simulink subsystem "rigid_body_sixdof"  (R2024b)
settings: Solver=VariableStepAuto  StartTime=0.0  StopTime=10.0  RelTol=1e-3
model mask{pos_0=[0; 0; 0], vel_0=[0; 0; 0], ornt_0=[1; 0; 0; 0], mass=1, inertia=eye(2), spin_0=[0; 0; 0]}
  mask prompts: pos_0 "Initial position, inertial [m]"; vel_0 "Initial velocity, inertial [m/s]"; ornt_0 "Initial orientation [quat]"; mass "Constant mass"; inertia "Rotational inertia, body coordinates"; spin_0 "Initial spin [rad/s]"
settings Model: Creator=yevge  LastModifiedBy=Yevgeniy Gorbachev

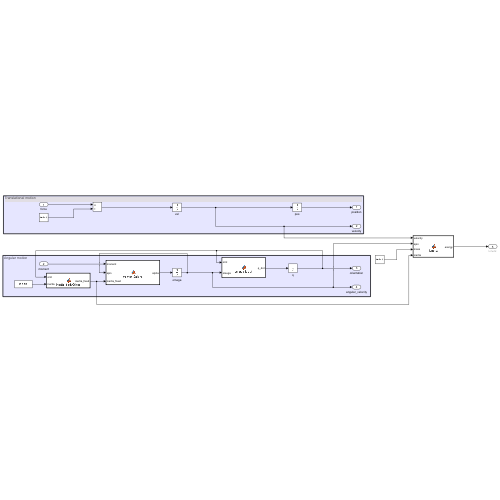
[thumbnail: Simulink's stored preview of the top-level diagram]
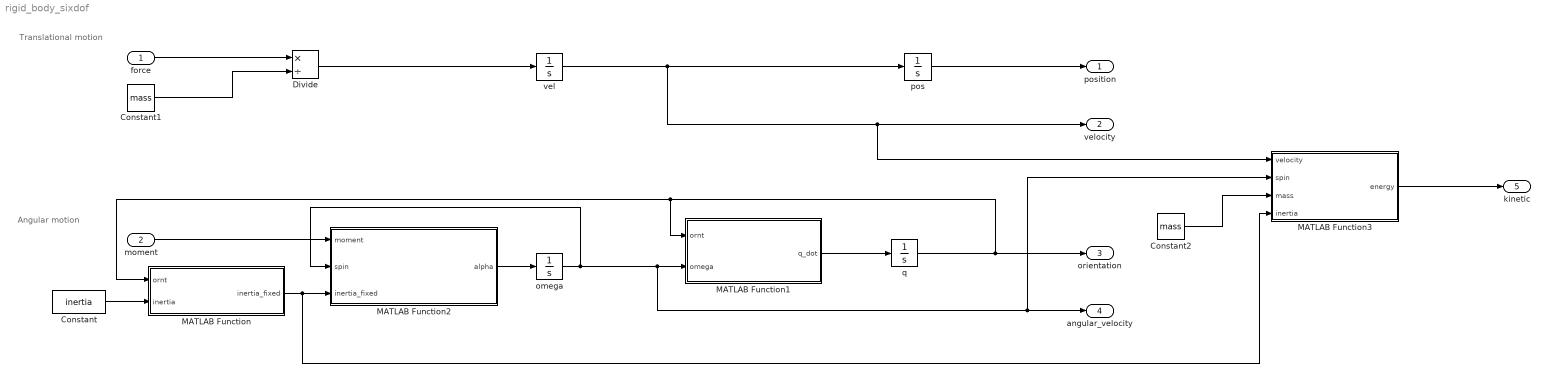
== system rigid_body_sixdof ==
  note: Angular motion
  note: Translational motion
  force : Inport  Unit=N  PortDimensions=[3 1]
  moment : Inport  Port=2  Unit=N*m@torque  PortDimensions=[3 1]
  Constant : Constant  Value=inertia
  Constant1 : Constant  Value=mass
  Constant2 : Constant  Value=mass
  Divide : Product  Inputs=*/
  MATLAB Function : MATLAB Function  TreatAsAtomicUnit=on
  MATLAB Function1 : MATLAB Function  TreatAsAtomicUnit=on
  MATLAB Function2 : MATLAB Function  TreatAsAtomicUnit=on
  MATLAB Function3 : MATLAB Function  TreatAsAtomicUnit=on
  omega : Integrator  InitialCondition=spin_0  ContinuousStateAttributes='angular_velocity'
  pos : Integrator  InitialCondition=pos_0  ContinuousStateAttributes='position'
  q : Integrator  InitialCondition=ornt_0  ContinuousStateAttributes='orientation'
  vel : Integrator  InitialCondition=vel_0  ContinuousStateAttributes='velocity'
  position : Outport  Unit=m  PortDimensions=[3 1]
  velocity : Outport  Port=2  Unit=m/s  PortDimensions=[3 1]
  orientation : Outport  Port=3  Unit=1  PortDimensions=[4 1]
  angular_velocity : Outport  Port=4  Unit=rad/s  PortDimensions=[3 1]
  kinetic : Outport  Port=5  Unit=J  PortDimensions=1
  wires:
  MATLAB Function1/1(q_dot) -> q/1
  q/1 -> orientation/1, MATLAB Function1/1(ornt), MATLAB Function/1(ornt)
  force/1 -> Divide/1
  Divide/1 -> vel/1
  vel/1 -> MATLAB Function3/1(velocity), velocity/1, pos/1
  pos/1 -> position/1
  MATLAB Function3/1(energy) -> kinetic/1
  MATLAB Function2/1(alpha) -> omega/1
  MATLAB Function/1(inertia_fixed) -> MATLAB Function3/4(inertia), MATLAB Function2/3(inertia_fixed)
  Constant1/1 -> Divide/2
  moment/1 -> MATLAB Function2/1(moment)
  Constant/1 -> MATLAB Function/2(inertia)
  Constant2/1 -> MATLAB Function3/3(mass)
  omega/1 -> MATLAB Function3/2(spin), angular_velocity/1, MATLAB Function1/2(omega), MATLAB Function2/2(spin)

== matlab function rigid_body_sixdof/MATLAB Function1 ==
  data: ornt input size=[4 1]; omega input size=[3 1]; q_dot output size=[4 1]
function q_dot = omega2qdot(ornt, omega)
    q_dot = 0.5*quatmultiply([0; omega]', ornt')';
end

== matlab function rigid_body_sixdof/MATLAB Function ==
  data: inertia_fixed output size=[3 3]; ornt input size=[4 1]; inertia input double size=[3 3]
function inertia_fixed = inertia_body2fixed(ornt, inertia)
    direction = quat2dcm(ornt');
    inertia_fixed = direction.' * inertia * direction;
end

== matlab function rigid_body_sixdof/MATLAB Function2 ==
  data: moment input size=[3 1]; alpha output size=[3 1]; spin input size=[3 1]; inertia_fixed input size=[3 3]
function alpha = moment2alpha(moment, spin, inertia_fixed)
        alpha = inertia_fixed \ (moment - cross(spin, inertia_fixed*spin));
end

== matlab function rigid_body_sixdof/MATLAB Function3 ==
  data: velocity input; energy output; spin input; mass input; inertia input
function energy = kinetic(velocity, spin, mass, inertia)
    tkinetic = 0.5 * mass * dot(velocity, velocity);
    rkinetic = 0.5 * dot(spin, inertia * spin);
    energy = tkinetic + rkinetic;
end
